simulink model "W2_Problem_1"  (R2020a)
settings: Solver=VariableStepAuto  StartTime=0.0  StopTime=10.0  RelTol=1e-3
settings Model: Creator=user  LastModifiedBy=user

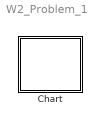
== system W2_Problem_1 ==
  Chart : Stateflow chart  TreatAsAtomicUnit=on

== stateflow chart W2_Problem_1/Chart ==
  state State_000
  state State_001
  state State_010
  state State_100
  state State_011
  (default) -> State_000
